simulink model "TorqueVect"  (Simulink 10.1)
settings: Solver=ode45  StartTime=0.0  StopTime=inf  RelTol=1e-3  EnableMultiTasking=on
undefined symbols (not defined in the file or in its folder): TC_Decr_Gas, TC_Derivative, TC_Incr_Gas, TC_On, TC_Relay_Off, TC_Relay_On, TV_On, TV_Override
libraries: CarMaker4SL x33, simulink x5, simulink_extras x4
(part 3 of 3)

== system TorqueVect/CarMaker/IPG Vehicle/PowerTrain/PTControl Example/PTControl_In/CreateBus PTC GearBoxM_In1 ==
  In : Inport
  BusCreator : BusCreator  Inputs=20
  Demux : Demux  Outputs=20
      settings: DisplayOption=none
  Out : Outport  VectorParamsAs1DForOutWhenUnconnected=off
  wires:
  In/1 -> Demux/1
  BusCreator/1 -> Out/1
  Demux/1 -> BusCreator/1  "PTC GearBoxM_In1 GearNo"
  Demux/2 -> BusCreator/2  "PTC GearBoxM_In1 GearNo_dis"
  Demux/3 -> BusCreator/3  "PTC GearBoxM_In1 Trq_DriveSrc_trg"
  Demux/4 -> BusCreator/4  "PTC GearBoxM_In1 i"
  Demux/5 -> BusCreator/5  "PTC GearBoxM_In1 rotv_in"
  Demux/6 -> BusCreator/6  "PTC GearBoxM_In1 rotv_out"
  Demux/7 -> BusCreator/7  "PTC GearBoxM_In1 Trq_in"
  Demux/8 -> BusCreator/8  "PTC GearBoxM_In1 Trq_out"
  Demux/9 -> BusCreator/9  "PTC GearBoxM_In1 Clutch Pos"
  Demux/10 -> BusCreator/10  "PTC GearBoxM_In1 Clutch rotv_in"
  Demux/11 -> BusCreator/11  "PTC GearBoxM_In1 Clutch rotv_out"
  Demux/12 -> BusCreator/12  "PTC GearBoxM_In1 Clutch Trq_in"
  Demux/13 -> BusCreator/13  "PTC GearBoxM_In1 Clutch Trq_out"
  Demux/14 -> BusCreator/14  "PTC GearBoxM_In1 Clutch i_TrqIn2Out"
  Demux/15 -> BusCreator/15  "PTC GearBoxM_In1 Clutch_dis Pos"
  Demux/16 -> BusCreator/16  "PTC GearBoxM_In1 Clutch_dis rotv_in"
  Demux/17 -> BusCreator/17  "PTC GearBoxM_In1 Clutch_dis rotv_out"
  Demux/18 -> BusCreator/18  "PTC GearBoxM_In1 Clutch_dis Trq_in"
  Demux/19 -> BusCreator/19  "PTC GearBoxM_In1 Clutch_dis Trq_out"
  Demux/20 -> BusCreator/20  "PTC GearBoxM_In1 Clutch_dis i_TrqIn2Out"

== system TorqueVect/CarMaker/IPG Vehicle/PowerTrain/PTControl Example/PTControl_In/CreateBus PTC GearBoxM_In2 ==
  In : Inport
  BusCreator : BusCreator  Inputs=20
  Demux : Demux  Outputs=20
      settings: DisplayOption=none
  Out : Outport  VectorParamsAs1DForOutWhenUnconnected=off
  wires:
  In/1 -> Demux/1
  BusCreator/1 -> Out/1
  Demux/1 -> BusCreator/1  "PTC GearBoxM_In2 GearNo"
  Demux/2 -> BusCreator/2  "PTC GearBoxM_In2 GearNo_dis"
  Demux/3 -> BusCreator/3  "PTC GearBoxM_In2 Trq_DriveSrc_trg"
  Demux/4 -> BusCreator/4  "PTC GearBoxM_In2 i"
  Demux/5 -> BusCreator/5  "PTC GearBoxM_In2 rotv_in"
  Demux/6 -> BusCreator/6  "PTC GearBoxM_In2 rotv_out"
  Demux/7 -> BusCreator/7  "PTC GearBoxM_In2 Trq_in"
  Demux/8 -> BusCreator/8  "PTC GearBoxM_In2 Trq_out"
  Demux/9 -> BusCreator/9  "PTC GearBoxM_In2 Clutch Pos"
  Demux/10 -> BusCreator/10  "PTC GearBoxM_In2 Clutch rotv_in"
  Demux/11 -> BusCreator/11  "PTC GearBoxM_In2 Clutch rotv_out"
  Demux/12 -> BusCreator/12  "PTC GearBoxM_In2 Clutch Trq_in"
  Demux/13 -> BusCreator/13  "PTC GearBoxM_In2 Clutch Trq_out"
  Demux/14 -> BusCreator/14  "PTC GearBoxM_In2 Clutch i_TrqIn2Out"
  Demux/15 -> BusCreator/15  "PTC GearBoxM_In2 Clutch_dis Pos"
  Demux/16 -> BusCreator/16  "PTC GearBoxM_In2 Clutch_dis rotv_in"
  Demux/17 -> BusCreator/17  "PTC GearBoxM_In2 Clutch_dis rotv_out"
  Demux/18 -> BusCreator/18  "PTC GearBoxM_In2 Clutch_dis Trq_in"
  Demux/19 -> BusCreator/19  "PTC GearBoxM_In2 Clutch_dis Trq_out"
  Demux/20 -> BusCreator/20  "PTC GearBoxM_In2 Clutch_dis i_TrqIn2Out"

== system TorqueVect/CarMaker/IPG Vehicle/PowerTrain/PTControl Example/PTControl_In/CreateBus PTC GearBoxM_In3 ==
  In : Inport
  BusCreator : BusCreator  Inputs=20
  Demux : Demux  Outputs=20
      settings: DisplayOption=none
  Out : Outport  VectorParamsAs1DForOutWhenUnconnected=off
  wires:
  In/1 -> Demux/1
  BusCreator/1 -> Out/1
  Demux/1 -> BusCreator/1  "PTC GearBoxM_In3 GearNo"
  Demux/2 -> BusCreator/2  "PTC GearBoxM_In3 GearNo_dis"
  Demux/3 -> BusCreator/3  "PTC GearBoxM_In3 Trq_DriveSrc_trg"
  Demux/4 -> BusCreator/4  "PTC GearBoxM_In3 i"
  Demux/5 -> BusCreator/5  "PTC GearBoxM_In3 rotv_in"
  Demux/6 -> BusCreator/6  "PTC GearBoxM_In3 rotv_out"
  Demux/7 -> BusCreator/7  "PTC GearBoxM_In3 Trq_in"
  Demux/8 -> BusCreator/8  "PTC GearBoxM_In3 Trq_out"
  Demux/9 -> BusCreator/9  "PTC GearBoxM_In3 Clutch Pos"
  Demux/10 -> BusCreator/10  "PTC GearBoxM_In3 Clutch rotv_in"
  Demux/11 -> BusCreator/11  "PTC GearBoxM_In3 Clutch rotv_out"
  Demux/12 -> BusCreator/12  "PTC GearBoxM_In3 Clutch Trq_in"
  Demux/13 -> BusCreator/13  "PTC GearBoxM_In3 Clutch Trq_out"
  Demux/14 -> BusCreator/14  "PTC GearBoxM_In3 Clutch i_TrqIn2Out"
  Demux/15 -> BusCreator/15  "PTC GearBoxM_In3 Clutch_dis Pos"
  Demux/16 -> BusCreator/16  "PTC GearBoxM_In3 Clutch_dis rotv_in"
  Demux/17 -> BusCreator/17  "PTC GearBoxM_In3 Clutch_dis rotv_out"
  Demux/18 -> BusCreator/18  "PTC GearBoxM_In3 Clutch_dis Trq_in"
  Demux/19 -> BusCreator/19  "PTC GearBoxM_In3 Clutch_dis Trq_out"
  Demux/20 -> BusCreator/20  "PTC GearBoxM_In3 Clutch_dis i_TrqIn2Out"

== system TorqueVect/CarMaker/IPG Vehicle/PowerTrain/PTControl Example/PTControl_In/CreateBus PTC ISGIn ==
  In : Inport
  BusCreator : BusCreator  Inputs=9
  Demux : Demux  Outputs=9
      settings: DisplayOption=none
  Out : Outport  VectorParamsAs1DForOutWhenUnconnected=off
  wires:
  In/1 -> Demux/1
  BusCreator/1 -> Out/1
  Demux/1 -> BusCreator/1  "PTC ISGIn rotv"
  Demux/2 -> BusCreator/2  "PTC ISGIn Trq"
  Demux/3 -> BusCreator/3  "PTC ISGIn TrqMot_max"
  Demux/4 -> BusCreator/4  "PTC ISGIn TrqGen_max"
  Demux/5 -> BusCreator/5  "PTC ISGIn PwrElec"
  Demux/6 -> BusCreator/6  "PTC ISGIn i_M2W_FL"
  Demux/7 -> BusCreator/7  "PTC ISGIn i_M2W_FR"
  Demux/8 -> BusCreator/8  "PTC ISGIn i_M2W_RL"
  Demux/9 -> BusCreator/9  "PTC ISGIn i_M2W_RR"

== system TorqueVect/CarMaker/IPG Vehicle/PowerTrain/PTControl Example/PTControl_In/CreateBus PTC MotorIn0 ==
  In : Inport
  BusCreator : BusCreator  Inputs=9
  Demux : Demux  Outputs=9
      settings: DisplayOption=none
  Out : Outport  VectorParamsAs1DForOutWhenUnconnected=off
  wires:
  In/1 -> Demux/1
  BusCreator/1 -> Out/1
  Demux/1 -> BusCreator/1  "PTC MotorIn0 rotv"
  Demux/2 -> BusCreator/2  "PTC MotorIn0 Trq"
  Demux/3 -> BusCreator/3  "PTC MotorIn0 TrqMot_max"
  Demux/4 -> BusCreator/4  "PTC MotorIn0 TrqGen_max"
  Demux/5 -> BusCreator/5  "PTC MotorIn0 PwrElec"
  Demux/6 -> BusCreator/6  "PTC MotorIn0 i_M2W_FL"
  Demux/7 -> BusCreator/7  "PTC MotorIn0 i_M2W_FR"
  Demux/8 -> BusCreator/8  "PTC MotorIn0 i_M2W_RL"
  Demux/9 -> BusCreator/9  "PTC MotorIn0 i_M2W_RR"

== system TorqueVect/CarMaker/IPG Vehicle/PowerTrain/PTControl Example/PTControl_In/CreateBus PTC MotorIn1 ==
  In : Inport
  BusCreator : BusCreator  Inputs=9
  Demux : Demux  Outputs=9
      settings: DisplayOption=none
  Out : Outport  VectorParamsAs1DForOutWhenUnconnected=off
  wires:
  In/1 -> Demux/1
  BusCreator/1 -> Out/1
  Demux/1 -> BusCreator/1  "PTC MotorIn1 rotv"
  Demux/2 -> BusCreator/2  "PTC MotorIn1 Trq"
  Demux/3 -> BusCreator/3  "PTC MotorIn1 TrqMot_max"
  Demux/4 -> BusCreator/4  "PTC MotorIn1 TrqGen_max"
  Demux/5 -> BusCreator/5  "PTC MotorIn1 PwrElec"
  Demux/6 -> BusCreator/6  "PTC MotorIn1 i_M2W_FL"
  Demux/7 -> BusCreator/7  "PTC MotorIn1 i_M2W_FR"
  Demux/8 -> BusCreator/8  "PTC MotorIn1 i_M2W_RL"
  Demux/9 -> BusCreator/9  "PTC MotorIn1 i_M2W_RR"

== system TorqueVect/CarMaker/IPG Vehicle/PowerTrain/PTControl Example/PTControl_In/CreateBus PTC MotorIn2 ==
  In : Inport
  BusCreator : BusCreator  Inputs=9
  Demux : Demux  Outputs=9
      settings: DisplayOption=none
  Out : Outport  VectorParamsAs1DForOutWhenUnconnected=off
  wires:
  In/1 -> Demux/1
  BusCreator/1 -> Out/1
  Demux/1 -> BusCreator/1  "PTC MotorIn2 rotv"
  Demux/2 -> BusCreator/2  "PTC MotorIn2 Trq"
  Demux/3 -> BusCreator/3  "PTC MotorIn2 TrqMot_max"
  Demux/4 -> BusCreator/4  "PTC MotorIn2 TrqGen_max"
  Demux/5 -> BusCreator/5  "PTC MotorIn2 PwrElec"
  Demux/6 -> BusCreator/6  "PTC MotorIn2 i_M2W_FL"
  Demux/7 -> BusCreator/7  "PTC MotorIn2 i_M2W_FR"
  Demux/8 -> BusCreator/8  "PTC MotorIn2 i_M2W_RL"
  Demux/9 -> BusCreator/9  "PTC MotorIn2 i_M2W_RR"

== system TorqueVect/CarMaker/IPG Vehicle/PowerTrain/PTControl Example/PTControl_In/CreateBus PTC MotorIn3 ==
  In : Inport
  BusCreator : BusCreator  Inputs=9
  Demux : Demux  Outputs=9
      settings: DisplayOption=none
  Out : Outport  VectorParamsAs1DForOutWhenUnconnected=off
  wires:
  In/1 -> Demux/1
  BusCreator/1 -> Out/1
  Demux/1 -> BusCreator/1  "PTC MotorIn3 rotv"
  Demux/2 -> BusCreator/2  "PTC MotorIn3 Trq"
  Demux/3 -> BusCreator/3  "PTC MotorIn3 TrqMot_max"
  Demux/4 -> BusCreator/4  "PTC MotorIn3 TrqGen_max"
  Demux/5 -> BusCreator/5  "PTC MotorIn3 PwrElec"
  Demux/6 -> BusCreator/6  "PTC MotorIn3 i_M2W_FL"
  Demux/7 -> BusCreator/7  "PTC MotorIn3 i_M2W_FR"
  Demux/8 -> BusCreator/8  "PTC MotorIn3 i_M2W_RL"
  Demux/9 -> BusCreator/9  "PTC MotorIn3 i_M2W_RR"

== system TorqueVect/CarMaker/IPG Vehicle/PowerTrain/PTControl Example/PTControl_In/CreateBus PTC PwrSupplyIn ==
  In : Inport
  BusCreator : BusCreator  Inputs=12
  Demux : Demux  Outputs=12
      settings: DisplayOption=none
  Out : Outport  VectorParamsAs1DForOutWhenUnconnected=off
  wires:
  In/1 -> Demux/1
  BusCreator/1 -> Out/1
  Demux/1 -> BusCreator/1  "PTC PwrSupplyIn Pwr_LV"
  Demux/2 -> BusCreator/2  "PTC PwrSupplyIn Pwr_HV1"
  Demux/3 -> BusCreator/3  "PTC PwrSupplyIn Pwr_HV2"
  Demux/4 -> BusCreator/4  "PTC PwrSupplyIn Voltage_LV"
  Demux/5 -> BusCreator/5  "PTC PwrSupplyIn Voltage_HV1"
  Demux/6 -> BusCreator/6  "PTC PwrSupplyIn Voltage_HV2"
  Demux/7 -> BusCreator/7  "PTC PwrSupplyIn Pwr_HV1toLV"
  Demux/8 -> BusCreator/8  "PTC PwrSupplyIn Pwr_HV1toHV2"
  Demux/9 -> BusCreator/9  "PTC PwrSupplyIn Pwr_HV1toLV_max"
  Demux/10 -> BusCreator/10  "PTC PwrSupplyIn Pwr_HV1toHV2_max"
  Demux/11 -> BusCreator/11  "PTC PwrSupplyIn Eta_HV1toLV"
  Demux/12 -> BusCreator/12  "PTC PwrSupplyIn Eta_HV1toHV2"

== system TorqueVect/CarMaker/IPG Vehicle/PowerTrain/PTControl Example/PTControl_In/CreateBus PTC Vehicle Ctrl ==
  In : Inport
  BusCreator : BusCreator  Inputs=8
  Demux : Demux  Outputs=8
      settings: DisplayOption=none
  Out : Outport  VectorParamsAs1DForOutWhenUnconnected=off
  wires:
  In/1 -> Demux/1
  BusCreator/1 -> Out/1
  Demux/1 -> BusCreator/1  "PTC Key"
  Demux/2 -> BusCreator/2  "PTC SST"
  Demux/3 -> BusCreator/3  "PTC SelectorCtrl"
  Demux/4 -> BusCreator/4  "PTC GearNoTrg"
  Demux/5 -> BusCreator/5  "PTC Clutch"
  Demux/6 -> BusCreator/6  "PTC Gas"
  Demux/7 -> BusCreator/7  "PTC Brake"
  Demux/8 -> BusCreator/8  "PTC Velocity"

== system TorqueVect/CarMaker/IPG Vehicle/PowerTrain/PTControl Example/PTControl_In/CreateBus PTC WheelIn ==
  In : Inport
  BusCreator : BusCreator  Inputs=4
  Demux : Demux
      settings: DisplayOption=none
  Out : Outport  VectorParamsAs1DForOutWhenUnconnected=off
  wires:
  In/1 -> Demux/1
  BusCreator/1 -> Out/1
  Demux/1 -> BusCreator/1  "PTC WheelIn_FL Trq_BrakeReg_trg"
  Demux/2 -> BusCreator/2  "PTC WheelIn_FR Trq_BrakeReg_trg"
  Demux/3 -> BusCreator/3  "PTC WheelIn_RL Trq_BrakeReg_trg"
  Demux/4 -> BusCreator/4  "PTC WheelIn_RR Trq_BrakeReg_trg"

== system TorqueVect/CarMaker/IPG Vehicle/PowerTrain/PTControl Example/PTControl_In/CreateBus PTC_Cfg Battery ==
  In : Inport
  BusCreator : BusCreator  Inputs=8
  Demux : Demux  Outputs=8
      settings: DisplayOption=none
  Out : Outport  VectorParamsAs1DForOutWhenUnconnected=off
  wires:
  In/1 -> Demux/1
  BusCreator/1 -> Out/1
  Demux/1 -> BusCreator/1  "PTC_Cfg BattLV SOC_min"
  Demux/2 -> BusCreator/2  "PTC_Cfg BattLV SOC_max"
  Demux/3 -> BusCreator/3  "PTC_Cfg BattLV Capacity"
  Demux/4 -> BusCreator/4  "PTC_Cfg BattLV Voltage"
  Demux/5 -> BusCreator/5  "PTC_Cfg BattHV SOC_min"
  Demux/6 -> BusCreator/6  "PTC_Cfg BattHV SOC_max"
  Demux/7 -> BusCreator/7  "PTC_Cfg BattHV Capacity"
  Demux/8 -> BusCreator/8  "PTC_Cfg BattHV Voltage"

== system TorqueVect/CarMaker/IPG Vehicle/PowerTrain/PTControl Example/PTControl_In/CreateBus PTC_Cfg Engine ==
  In : Inport
  BusCreator : BusCreator  Inputs=4
  Demux : Demux
      settings: DisplayOption=none
  Out : Outport  VectorParamsAs1DForOutWhenUnconnected=off
  wires:
  In/1 -> Demux/1
  BusCreator/1 -> Out/1
  Demux/1 -> BusCreator/1  "PTC_Cfg Engine Fuel_l2kWh"
  Demux/2 -> BusCreator/2  "PTC_Cfg Engine rotv_max"
  Demux/3 -> BusCreator/3  "PTC_Cfg Engine rotv_idle"
  Demux/4 -> BusCreator/4  "PTC_Cfg Engine rotv_opt"

== system TorqueVect/CarMaker/IPG Vehicle/PowerTrain/PTControl Example/PTControl_In/CreateBus PTC_Cfg GearBox ==
  In : Inport
  BusCreator : BusCreator  Inputs=38
  Demux : Demux  Outputs=38
      settings: DisplayOption=none
  Out : Outport  VectorParamsAs1DForOutWhenUnconnected=off
  wires:
  In/1 -> Demux/1
  BusCreator/1 -> Out/1
  Demux/1 -> BusCreator/1  "PTC_Cfg GearBox GBKind"
  Demux/2 -> BusCreator/2  "PTC_Cfg GearBox ClKind"
  Demux/3 -> BusCreator/3  "PTC_Cfg GearBox nFGears"
  Demux/4 -> BusCreator/4  "PTC_Cfg GearBox iFGear0"
  Demux/5 -> BusCreator/5  "PTC_Cfg GearBox iFGear1"
  Demux/6 -> BusCreator/6  "PTC_Cfg GearBox iFGear2"
  Demux/7 -> BusCreator/7  "PTC_Cfg GearBox iFGear3"
  Demux/8 -> BusCreator/8  "PTC_Cfg GearBox iFGear4"
  Demux/9 -> BusCreator/9  "PTC_Cfg GearBox iFGear5"
  Demux/10 -> BusCreator/10  "PTC_Cfg GearBox iFGear6"
  Demux/11 -> BusCreator/11  "PTC_Cfg GearBox iFGear7"
  Demux/12 -> BusCreator/12  "PTC_Cfg GearBox iFGear8"
  Demux/13 -> BusCreator/13  "PTC_Cfg GearBox iFGear9"
  Demux/14 -> BusCreator/14  "PTC_Cfg GearBox iFGear10"
  Demux/15 -> BusCreator/15  "PTC_Cfg GearBox iFGear11"
  Demux/16 -> BusCreator/16  "PTC_Cfg GearBox iFGear12"
  Demux/17 -> BusCreator/17  "PTC_Cfg GearBox iFGear13"
  Demux/18 -> BusCreator/18  "PTC_Cfg GearBox iFGear14"
  Demux/19 -> BusCreator/19  "PTC_Cfg GearBox iFGear15"
  Demux/20 -> BusCreator/20  "PTC_Cfg GearBox iFGear16"
  Demux/21 -> BusCreator/21  "PTC_Cfg GearBox nBGears"
  Demux/22 -> BusCreator/22  "PTC_Cfg GearBox iBGear0"
  Demux/23 -> BusCreator/23  "PTC_Cfg GearBox iBGear1"
  Demux/24 -> BusCreator/24  "PTC_Cfg GearBox iBGear2"
  Demux/25 -> BusCreator/25  "PTC_Cfg GearBox iBGear3"
  Demux/26 -> BusCreator/26  "PTC_Cfg GearBox iBGear4"
  Demux/27 -> BusCreator/27  "PTC_Cfg GearBox iBGear5"
  Demux/28 -> BusCreator/28  "PTC_Cfg GearBox iBGear6"
  Demux/29 -> BusCreator/29  "PTC_Cfg GearBox iBGear7"
  Demux/30 -> BusCreator/30  "PTC_Cfg GearBox iBGear8"
  Demux/31 -> BusCreator/31  "PTC_Cfg GearBox iBGear9"
  Demux/32 -> BusCreator/32  "PTC_Cfg GearBox iBGear10"
  Demux/33 -> BusCreator/33  "PTC_Cfg GearBox iBGear11"
  Demux/34 -> BusCreator/34  "PTC_Cfg GearBox iBGear12"
  Demux/35 -> BusCreator/35  "PTC_Cfg GearBox iBGear13"
  Demux/36 -> BusCreator/36  "PTC_Cfg GearBox iBGear14"
  Demux/37 -> BusCreator/37  "PTC_Cfg GearBox iBGear15"
  Demux/38 -> BusCreator/38  "PTC_Cfg GearBox iBGear16"

== system TorqueVect/CarMaker/IPG Vehicle/PowerTrain/PTControl Example/PTControl_In/CreateBus PTC_Cfg GearBoxM0 ==
  In : Inport
  BusCreator : BusCreator  Inputs=38
  Demux : Demux  Outputs=38
      settings: DisplayOption=none
  Out : Outport  VectorParamsAs1DForOutWhenUnconnected=off
  wires:
  In/1 -> Demux/1
  BusCreator/1 -> Out/1
  Demux/1 -> BusCreator/1  "PTC_Cfg GearBoxM0 GBKind"
  Demux/2 -> BusCreator/2  "PTC_Cfg GearBoxM0 ClKind"
  Demux/3 -> BusCreator/3  "PTC_Cfg GearBoxM0 nFGears"
  Demux/4 -> BusCreator/4  "PTC_Cfg GearBoxM0 iFGear0"
  Demux/5 -> BusCreator/5  "PTC_Cfg GearBoxM0 iFGear1"
  Demux/6 -> BusCreator/6  "PTC_Cfg GearBoxM0 iFGear2"
  Demux/7 -> BusCreator/7  "PTC_Cfg GearBoxM0 iFGear3"
  Demux/8 -> BusCreator/8  "PTC_Cfg GearBoxM0 iFGear4"
  Demux/9 -> BusCreator/9  "PTC_Cfg GearBoxM0 iFGear5"
  Demux/10 -> BusCreator/10  "PTC_Cfg GearBoxM0 iFGear6"
  Demux/11 -> BusCreator/11  "PTC_Cfg GearBoxM0 iFGear7"
  Demux/12 -> BusCreator/12  "PTC_Cfg GearBoxM0 iFGear8"
  Demux/13 -> BusCreator/13  "PTC_Cfg GearBoxM0 iFGear9"
  Demux/14 -> BusCreator/14  "PTC_Cfg GearBoxM0 iFGear10"
  Demux/15 -> BusCreator/15  "PTC_Cfg GearBoxM0 iFGear11"
  Demux/16 -> BusCreator/16  "PTC_Cfg GearBoxM0 iFGear12"
  Demux/17 -> BusCreator/17  "PTC_Cfg GearBoxM0 iFGear13"
  Demux/18 -> BusCreator/18  "PTC_Cfg GearBoxM0 iFGear14"
  Demux/19 -> BusCreator/19  "PTC_Cfg GearBoxM0 iFGear15"
  Demux/20 -> BusCreator/20  "PTC_Cfg GearBoxM0 iFGear16"
  Demux/21 -> BusCreator/21  "PTC_Cfg GearBoxM0 nBGears"
  Demux/22 -> BusCreator/22  "PTC_Cfg GearBoxM0 iBGear0"
  Demux/23 -> BusCreator/23  "PTC_Cfg GearBoxM0 iBGear1"
  Demux/24 -> BusCreator/24  "PTC_Cfg GearBoxM0 iBGear2"
  Demux/25 -> BusCreator/25  "PTC_Cfg GearBoxM0 iBGear3"
  Demux/26 -> BusCreator/26  "PTC_Cfg GearBoxM0 iBGear4"
  Demux/27 -> BusCreator/27  "PTC_Cfg GearBoxM0 iBGear5"
  Demux/28 -> BusCreator/28  "PTC_Cfg GearBoxM0 iBGear6"
  Demux/29 -> BusCreator/29  "PTC_Cfg GearBoxM0 iBGear7"
  Demux/30 -> BusCreator/30  "PTC_Cfg GearBoxM0 iBGear8"
  Demux/31 -> BusCreator/31  "PTC_Cfg GearBoxM0 iBGear9"
  Demux/32 -> BusCreator/32  "PTC_Cfg GearBoxM0 iBGear10"
  Demux/33 -> BusCreator/33  "PTC_Cfg GearBoxM0 iBGear11"
  Demux/34 -> BusCreator/34  "PTC_Cfg GearBoxM0 iBGear12"
  Demux/35 -> BusCreator/35  "PTC_Cfg GearBoxM0 iBGear13"
  Demux/36 -> BusCreator/36  "PTC_Cfg GearBoxM0 iBGear14"
  Demux/37 -> BusCreator/37  "PTC_Cfg GearBoxM0 iBGear15"
  Demux/38 -> BusCreator/38  "PTC_Cfg GearBoxM0 iBGear16"

== system TorqueVect/CarMaker/IPG Vehicle/PowerTrain/PTControl Example/PTControl_In/CreateBus PTC_Cfg GearBoxM1 ==
  In : Inport
  BusCreator : BusCreator  Inputs=38
  Demux : Demux  Outputs=38
      settings: DisplayOption=none
  Out : Outport  VectorParamsAs1DForOutWhenUnconnected=off
  wires:
  In/1 -> Demux/1
  BusCreator/1 -> Out/1
  Demux/1 -> BusCreator/1  "PTC_Cfg GearBoxM1 GBKind"
  Demux/2 -> BusCreator/2  "PTC_Cfg GearBoxM1 ClKind"
  Demux/3 -> BusCreator/3  "PTC_Cfg GearBoxM1 nFGears"
  Demux/4 -> BusCreator/4  "PTC_Cfg GearBoxM1 iFGear0"
  Demux/5 -> BusCreator/5  "PTC_Cfg GearBoxM1 iFGear1"
  Demux/6 -> BusCreator/6  "PTC_Cfg GearBoxM1 iFGear2"
  Demux/7 -> BusCreator/7  "PTC_Cfg GearBoxM1 iFGear3"
  Demux/8 -> BusCreator/8  "PTC_Cfg GearBoxM1 iFGear4"
  Demux/9 -> BusCreator/9  "PTC_Cfg GearBoxM1 iFGear5"
  Demux/10 -> BusCreator/10  "PTC_Cfg GearBoxM1 iFGear6"
  Demux/11 -> BusCreator/11  "PTC_Cfg GearBoxM1 iFGear7"
  Demux/12 -> BusCreator/12  "PTC_Cfg GearBoxM1 iFGear8"
  Demux/13 -> BusCreator/13  "PTC_Cfg GearBoxM1 iFGear9"
  Demux/14 -> BusCreator/14  "PTC_Cfg GearBoxM1 iFGear10"
  Demux/15 -> BusCreator/15  "PTC_Cfg GearBoxM1 iFGear11"
  Demux/16 -> BusCreator/16  "PTC_Cfg GearBoxM1 iFGear12"
  Demux/17 -> BusCreator/17  "PTC_Cfg GearBoxM1 iFGear13"
  Demux/18 -> BusCreator/18  "PTC_Cfg GearBoxM1 iFGear14"
  Demux/19 -> BusCreator/19  "PTC_Cfg GearBoxM1 iFGear15"
  Demux/20 -> BusCreator/20  "PTC_Cfg GearBoxM1 iFGear16"
  Demux/21 -> BusCreator/21  "PTC_Cfg GearBoxM1 nBGears"
  Demux/22 -> BusCreator/22  "PTC_Cfg GearBoxM1 iBGear0"
  Demux/23 -> BusCreator/23  "PTC_Cfg GearBoxM1 iBGear1"
  Demux/24 -> BusCreator/24  "PTC_Cfg GearBoxM1 iBGear2"
  Demux/25 -> BusCreator/25  "PTC_Cfg GearBoxM1 iBGear3"
  Demux/26 -> BusCreator/26  "PTC_Cfg GearBoxM1 iBGear4"
  Demux/27 -> BusCreator/27  "PTC_Cfg GearBoxM1 iBGear5"
  Demux/28 -> BusCreator/28  "PTC_Cfg GearBoxM1 iBGear6"
  Demux/29 -> BusCreator/29  "PTC_Cfg GearBoxM1 iBGear7"
  Demux/30 -> BusCreator/30  "PTC_Cfg GearBoxM1 iBGear8"
  Demux/31 -> BusCreator/31  "PTC_Cfg GearBoxM1 iBGear9"
  Demux/32 -> BusCreator/32  "PTC_Cfg GearBoxM1 iBGear10"
  Demux/33 -> BusCreator/33  "PTC_Cfg GearBoxM1 iBGear11"
  Demux/34 -> BusCreator/34  "PTC_Cfg GearBoxM1 iBGear12"
  Demux/35 -> BusCreator/35  "PTC_Cfg GearBoxM1 iBGear13"
  Demux/36 -> BusCreator/36  "PTC_Cfg GearBoxM1 iBGear14"
  Demux/37 -> BusCreator/37  "PTC_Cfg GearBoxM1 iBGear15"
  Demux/38 -> BusCreator/38  "PTC_Cfg GearBoxM1 iBGear16"

== system TorqueVect/CarMaker/IPG Vehicle/PowerTrain/PTControl Example/PTControl_In/CreateBus PTC_Cfg GearBoxM2 ==
  In : Inport
  BusCreator : BusCreator  Inputs=38
  Demux : Demux  Outputs=38
      settings: DisplayOption=none
  Out : Outport  VectorParamsAs1DForOutWhenUnconnected=off
  wires:
  In/1 -> Demux/1
  BusCreator/1 -> Out/1
  Demux/1 -> BusCreator/1  "PTC_Cfg GearBoxM2 GBKind"
  Demux/2 -> BusCreator/2  "PTC_Cfg GearBoxM2 ClKind"
  Demux/3 -> BusCreator/3  "PTC_Cfg GearBoxM2 nFGears"
  Demux/4 -> BusCreator/4  "PTC_Cfg GearBoxM2 iFGear0"
  Demux/5 -> BusCreator/5  "PTC_Cfg GearBoxM2 iFGear1"
  Demux/6 -> BusCreator/6  "PTC_Cfg GearBoxM2 iFGear2"
  Demux/7 -> BusCreator/7  "PTC_Cfg GearBoxM2 iFGear3"
  Demux/8 -> BusCreator/8  "PTC_Cfg GearBoxM2 iFGear4"
  Demux/9 -> BusCreator/9  "PTC_Cfg GearBoxM2 iFGear5"
  Demux/10 -> BusCreator/10  "PTC_Cfg GearBoxM2 iFGear6"
  Demux/11 -> BusCreator/11  "PTC_Cfg GearBoxM2 iFGear7"
  Demux/12 -> BusCreator/12  "PTC_Cfg GearBoxM2 iFGear8"
  Demux/13 -> BusCreator/13  "PTC_Cfg GearBoxM2 iFGear9"
  Demux/14 -> BusCreator/14  "PTC_Cfg GearBoxM2 iFGear10"
  Demux/15 -> BusCreator/15  "PTC_Cfg GearBoxM2 iFGear11"
  Demux/16 -> BusCreator/16  "PTC_Cfg GearBoxM2 iFGear12"
  Demux/17 -> BusCreator/17  "PTC_Cfg GearBoxM2 iFGear13"
  Demux/18 -> BusCreator/18  "PTC_Cfg GearBoxM2 iFGear14"
  Demux/19 -> BusCreator/19  "PTC_Cfg GearBoxM2 iFGear15"
  Demux/20 -> BusCreator/20  "PTC_Cfg GearBoxM2 iFGear16"
  Demux/21 -> BusCreator/21  "PTC_Cfg GearBoxM2 nBGears"
  Demux/22 -> BusCreator/22  "PTC_Cfg GearBoxM2 iBGear0"
  Demux/23 -> BusCreator/23  "PTC_Cfg GearBoxM2 iBGear1"
  Demux/24 -> BusCreator/24  "PTC_Cfg GearBoxM2 iBGear2"
  Demux/25 -> BusCreator/25  "PTC_Cfg GearBoxM2 iBGear3"
  Demux/26 -> BusCreator/26  "PTC_Cfg GearBoxM2 iBGear4"
  Demux/27 -> BusCreator/27  "PTC_Cfg GearBoxM2 iBGear5"
  Demux/28 -> BusCreator/28  "PTC_Cfg GearBoxM2 iBGear6"
  Demux/29 -> BusCreator/29  "PTC_Cfg GearBoxM2 iBGear7"
  Demux/30 -> BusCreator/30  "PTC_Cfg GearBoxM2 iBGear8"
  Demux/31 -> BusCreator/31  "PTC_Cfg GearBoxM2 iBGear9"
  Demux/32 -> BusCreator/32  "PTC_Cfg GearBoxM2 iBGear10"
  Demux/33 -> BusCreator/33  "PTC_Cfg GearBoxM2 iBGear11"
  Demux/34 -> BusCreator/34  "PTC_Cfg GearBoxM2 iBGear12"
  Demux/35 -> BusCreator/35  "PTC_Cfg GearBoxM2 iBGear13"
  Demux/36 -> BusCreator/36  "PTC_Cfg GearBoxM2 iBGear14"
  Demux/37 -> BusCreator/37  "PTC_Cfg GearBoxM2 iBGear15"
  Demux/38 -> BusCreator/38  "PTC_Cfg GearBoxM2 iBGear16"

== system TorqueVect/CarMaker/IPG Vehicle/PowerTrain/PTControl Example/PTControl_In/CreateBus PTC_Cfg GearBoxM3 ==
  In : Inport
  BusCreator : BusCreator  Inputs=38
  Demux : Demux  Outputs=38
      settings: DisplayOption=none
  Out : Outport  VectorParamsAs1DForOutWhenUnconnected=off
  wires:
  In/1 -> Demux/1
  BusCreator/1 -> Out/1
  Demux/1 -> BusCreator/1  "PTC_Cfg GearBoxM3 GBKind"
  Demux/2 -> BusCreator/2  "PTC_Cfg GearBoxM3 ClKind"
  Demux/3 -> BusCreator/3  "PTC_Cfg GearBoxM3 nFGears"
  Demux/4 -> BusCreator/4  "PTC_Cfg GearBoxM3 iFGear0"
  Demux/5 -> BusCreator/5  "PTC_Cfg GearBoxM3 iFGear1"
  Demux/6 -> BusCreator/6  "PTC_Cfg GearBoxM3 iFGear2"
  Demux/7 -> BusCreator/7  "PTC_Cfg GearBoxM3 iFGear3"
  Demux/8 -> BusCreator/8  "PTC_Cfg GearBoxM3 iFGear4"
  Demux/9 -> BusCreator/9  "PTC_Cfg GearBoxM3 iFGear5"
  Demux/10 -> BusCreator/10  "PTC_Cfg GearBoxM3 iFGear6"
  Demux/11 -> BusCreator/11  "PTC_Cfg GearBoxM3 iFGear7"
  Demux/12 -> BusCreator/12  "PTC_Cfg GearBoxM3 iFGear8"
  Demux/13 -> BusCreator/13  "PTC_Cfg GearBoxM3 iFGear9"
  Demux/14 -> BusCreator/14  "PTC_Cfg GearBoxM3 iFGear10"
  Demux/15 -> BusCreator/15  "PTC_Cfg GearBoxM3 iFGear11"
  Demux/16 -> BusCreator/16  "PTC_Cfg GearBoxM3 iFGear12"
  Demux/17 -> BusCreator/17  "PTC_Cfg GearBoxM3 iFGear13"
  Demux/18 -> BusCreator/18  "PTC_Cfg GearBoxM3 iFGear14"
  Demux/19 -> BusCreator/19  "PTC_Cfg GearBoxM3 iFGear15"
  Demux/20 -> BusCreator/20  "PTC_Cfg GearBoxM3 iFGear16"
  Demux/21 -> BusCreator/21  "PTC_Cfg GearBoxM3 nBGears"
  Demux/22 -> BusCreator/22  "PTC_Cfg GearBoxM3 iBGear0"
  Demux/23 -> BusCreator/23  "PTC_Cfg GearBoxM3 iBGear1"
  Demux/24 -> BusCreator/24  "PTC_Cfg GearBoxM3 iBGear2"
  Demux/25 -> BusCreator/25  "PTC_Cfg GearBoxM3 iBGear3"
  Demux/26 -> BusCreator/26  "PTC_Cfg GearBoxM3 iBGear4"
  Demux/27 -> BusCreator/27  "PTC_Cfg GearBoxM3 iBGear5"
  Demux/28 -> BusCreator/28  "PTC_Cfg GearBoxM3 iBGear6"
  Demux/29 -> BusCreator/29  "PTC_Cfg GearBoxM3 iBGear7"
  Demux/30 -> BusCreator/30  "PTC_Cfg GearBoxM3 iBGear8"
  Demux/31 -> BusCreator/31  "PTC_Cfg GearBoxM3 iBGear9"
  Demux/32 -> BusCreator/32  "PTC_Cfg GearBoxM3 iBGear10"
  Demux/33 -> BusCreator/33  "PTC_Cfg GearBoxM3 iBGear11"
  Demux/34 -> BusCreator/34  "PTC_Cfg GearBoxM3 iBGear12"
  Demux/35 -> BusCreator/35  "PTC_Cfg GearBoxM3 iBGear13"
  Demux/36 -> BusCreator/36  "PTC_Cfg GearBoxM3 iBGear14"
  Demux/37 -> BusCreator/37  "PTC_Cfg GearBoxM3 iBGear15"
  Demux/38 -> BusCreator/38  "PTC_Cfg GearBoxM3 iBGear16"

== system TorqueVect/CarMaker/IPG Vehicle/PowerTrain/PTControl Example/PTControl_In/CreateBus PTC_Cfg ISG ==
  In : Inport
  BusCreator : BusCreator  Inputs=4
  Demux : Demux
      settings: DisplayOption=none
  Out : Outport  VectorParamsAs1DForOutWhenUnconnected=off
  wires:
  In/1 -> Demux/1
  BusCreator/1 -> Out/1
  Demux/1 -> BusCreator/1  "PTC_Cfg ISG Level"
  Demux/2 -> BusCreator/2  "PTC_Cfg ISG Ratio"
  Demux/3 -> BusCreator/3  "PTC_Cfg ISG rotv_Mot_max"
  Demux/4 -> BusCreator/4  "PTC_Cfg ISG rotv_Gen_max"

== system TorqueVect/CarMaker/IPG Vehicle/PowerTrain/PTControl Example/PTControl_In/CreateBus PTC_Cfg Misc ==
  In : Inport
  BusCreator : BusCreator  Inputs=13
  Demux : Demux  Outputs=13
      settings: DisplayOption=none
  Out : Outport  VectorParamsAs1DForOutWhenUnconnected=off
  wires:
  In/1 -> Demux/1
  BusCreator/1 -> Out/1
  Demux/1 -> BusCreator/1  "PTC_Cfg PTKind"
  Demux/2 -> BusCreator/2  "PTC_Cfg ClKind"
  Demux/3 -> BusCreator/3  "PTC_Cfg nMotor"
  Demux/4 -> BusCreator/4  "PTC_Cfg nGearBoxM"
  Demux/5 -> BusCreator/5  "PTC_Cfg nPlanetGear"
  Demux/6 -> BusCreator/6  "PTC_Cfg Vehicle_nWheels"
  Demux/7 -> BusCreator/7  "PTC_Cfg WheelRadius"
  Demux/8 -> BusCreator/8  "PTC_Cfg Aero_Frcx"
  Demux/9 -> BusCreator/9  "PTC_Cfg DL_iDiff_mean"
  Demux/10 -> BusCreator/10  "PTC_Cfg DriveSourcePos0"
  Demux/11 -> BusCreator/11  "PTC_Cfg DriveSourcePos1"
  Demux/12 -> BusCreator/12  "PTC_Cfg DriveSourcePos2"
  Demux/13 -> BusCreator/13  "PTC_Cfg DriveSourcePos3"

== system TorqueVect/CarMaker/IPG Vehicle/PowerTrain/PTControl Example/PTControl_In/CreateBus PTC_Cfg Motor ==
  In : Inport
  BusCreator : BusCreator  Inputs=16
  Demux : Demux  Outputs=16
      settings: DisplayOption=none
  Out : Outport  VectorParamsAs1DForOutWhenUnconnected=off
  wires:
  In/1 -> Demux/1
  BusCreator/1 -> Out/1
  Demux/1 -> BusCreator/1  "PTC_Cfg Motor0 Level"
  Demux/2 -> BusCreator/2  "PTC_Cfg Motor0 Ratio"
  Demux/3 -> BusCreator/3  "PTC_Cfg Motor0 rotv_Mot_max"
  Demux/4 -> BusCreator/4  "PTC_Cfg Motor0 rotv_Gen_max"
  Demux/5 -> BusCreator/5  "PTC_Cfg Motor1 Level"
  Demux/6 -> BusCreator/6  "PTC_Cfg Motor1 Ratio"
  Demux/7 -> BusCreator/7  "PTC_Cfg Motor1 rotv_Mot_max"
  Demux/8 -> BusCreator/8  "PTC_Cfg Motor1 rotv_Gen_max"
  Demux/9 -> BusCreator/9  "PTC_Cfg Motor2 Level"
  Demux/10 -> BusCreator/10  "PTC_Cfg Motor2 Ratio"
  Demux/11 -> BusCreator/11  "PTC_Cfg Motor2 rotv_Mot_max"
  Demux/12 -> BusCreator/12  "PTC_Cfg Motor2 rotv_Gen_max"
  Demux/13 -> BusCreator/13  "PTC_Cfg Motor3 Level"
  Demux/14 -> BusCreator/14  "PTC_Cfg Motor3 Ratio"
  Demux/15 -> BusCreator/15  "PTC_Cfg Motor3 rotv_Mot_max"
  Demux/16 -> BusCreator/16  "PTC_Cfg Motor3 rotv_Gen_max"

== system TorqueVect/CarMaker/IPG Vehicle/PowerTrain/PTControl Example/PTControl_In/CreateBus PTC_Cfg PlanetGear ==
  In : Inport
  BusCreator : BusCreator  Inputs=1
  Demux : Demux  Outputs=1
      settings: DisplayOption=none
  Out : Outport  VectorParamsAs1DForOutWhenUnconnected=off
  wires:
  In/1 -> Demux/1
  BusCreator/1 -> Out/1
  Demux/1 -> BusCreator/1  "PTC_Cfg PlanetGear0 Ratio"

== system TorqueVect/CarMaker/IPG Vehicle/PowerTrain/PTControl Example/PTControl/Torque Control 0/Electronic Gas Pedal FL ==
  TV_On : Inport
  VC.Gas : Inport  Port=2
  Define CM Dict : CarMaker4SL/Define CM Dict  xname=E_Gas_FL  xmono=off  xtype=Double4  xdvaplace=None  xnstates=0  xfirststate=0  xinitial=0
  Read CM Dict : CarMaker4SL/Read CM Dict  xname=E_Gas_FL  xsync=off  xstime=Continuous
  Read CM Dict1 : CarMaker4SL/Read CM Dict  xname=Car.LongSlipFL  xsync=off  xstime=Continuous
  Switch : Switch  Criteria=u2 > Threshold
  Traction Control FL : Subsystem
  Write CM Dict : CarMaker4SL/Write CM Dict  xname=E_Gas_FL  xsync=off
  Motor_Gas_FL : Outport  VectorParamsAs1DForOutWhenUnconnected=off
  wires:
  Read CM Dict/1 -> Traction Control FL/2(E_Gas.)
  Read CM Dict1/1 -> Traction Control FL/3(Car.LongSlip)
  VC.Gas/1 -> Switch/3, Traction Control FL/1(VC.Gas)
  Switch/1 -> Motor_Gas_FL/1
  TV_On/1 -> Switch/2
  Traction Control FL/1(E_Gas) -> Switch/1, Write CM Dict/1

== system TorqueVect/CarMaker/IPG Vehicle/PowerTrain/PTControl Example/PTControl/Torque Control 0/Torque Vectoring FL ==
  Abs : Abs
  Abs2 : Abs
  Constant : Constant
  Divide : Product  Inputs=*/
  Gain : Gain  Gain=-1
  Gravity : Gain  Gain=9.81
  Lookup Table : Lookup  InputValues=[0,0.1,0.2,0.3,0.4,0.5,0.6,0.7,0.8,1,2,3,4]  Table=[0,0,0.05,0.1,0.2,0.3,0.4,0.5,0.6,0.7,1,1,1]
  Override : Gain  Gain=TV_Override
  Product : Product  RndMeth=Zero
  Read CM Dict : CarMaker4SL/Read CM Dict  xname=Car.muRoadFL  xsync=off  xstime=Continuous
  Read CM Dict1 : CarMaker4SL/Read CM Dict  xname=Car.v  xsync=off  xstime=Continuous
  Read CM Dict2 : CarMaker4SL/Read CM Dict  xname=Car.YawRate  xsync=off  xstime=Continuous
  Read CM Dict3 : CarMaker4SL/Read CM Dict  xname=VC.Steer.Ang  xsync=off  xstime=Continuous
  Subtract : Sum  Inputs=+-
  Switch : Switch  Criteria=u2 > Threshold
  TV FL : Outport  VectorParamsAs1DForOutWhenUnconnected=off
  wires:
  Gain/1 -> Lookup Table/1
  Abs2/1 -> Subtract/2
  Lookup Table/1 -> Product/2
  Read CM Dict3/1 -> Gain/1
  Product/1 -> TV FL/1
  Subtract/1 -> Product/1
  Read CM Dict2/1 -> Abs2/1
  Divide/1 -> Subtract/1
  Abs/1 -> Divide/2
  Switch/1 -> Abs/1
  Constant/1 -> Switch/3
  Read CM Dict1/1 -> Switch/2, Switch/1
  Override/1 -> Divide/1
  Gravity/1 -> Override/1
  Read CM Dict/1 -> Gravity/1

== system TorqueVect/CarMaker/IPG Vehicle/PowerTrain/PTControl Example/PTControl/Torque Control 1/Electronic Gas Pedal FR ==
  TV_On : Inport
  VC.Gas : Inport  Port=2
  Define CM Dict : CarMaker4SL/Define CM Dict  xname=E_Gas_FR  xmono=off  xtype=Double4  xdvaplace=None  xnstates=0  xfirststate=0  xinitial=0
  Read CM Dict : CarMaker4SL/Read CM Dict  xname=E_Gas_FR  xsync=off  xstime=Continuous
  Read CM Dict1 : CarMaker4SL/Read CM Dict  xname=Car.LongSlipFR  xsync=off  xstime=Continuous
  Switch : Switch  Criteria=u2 > Threshold
  Traction Control FR : Subsystem
  Write CM Dict : CarMaker4SL/Write CM Dict  xname=E_Gas_FR  xsync=off
  Motor_Gas_FR : Outport  VectorParamsAs1DForOutWhenUnconnected=off
  wires:
  Traction Control FR/1(E_Gas) -> Write CM Dict/1, Switch/1
  TV_On/1 -> Switch/2
  Switch/1 -> Motor_Gas_FR/1
  VC.Gas/1 -> Traction Control FR/1(VC.Gas), Switch/3
  Read CM Dict1/1 -> Traction Control FR/3(Car.LongSlip)
  Read CM Dict/1 -> Traction Control FR/2(E_Gas.)

== system TorqueVect/CarMaker/IPG Vehicle/PowerTrain/PTControl Example/PTControl/Torque Control 1/Torque Vectoring FR ==
  Abs : Abs
  Abs2 : Abs
  Constant : Constant
  Divide : Product  Inputs=*/
  Gain : Gain  Gain=-1
  Gravity : Gain  Gain=9.81
  Lookup Table : Lookup  InputValues=[0,0.1,0.2,0.3,0.4,0.5,0.6,0.7,0.8,1,2,3,4]  Table=[0,0,0.05,0.1,0.2,0.3,0.4,0.5,0.6,0.7,1,1,1]
  Override : Gain  Gain=TV_Override
  Product : Product  RndMeth=Zero
  Read CM Dict : CarMaker4SL/Read CM Dict  xname=Car.muRoadFR  xsync=off  xstime=Continuous
  Read CM Dict1 : CarMaker4SL/Read CM Dict  xname=Car.v  xsync=off  xstime=Continuous
  Read CM Dict2 : CarMaker4SL/Read CM Dict  xname=Car.YawRate  xsync=off  xstime=Continuous
  Read CM Dict3 : CarMaker4SL/Read CM Dict  xname=VC.Steer.Ang  xsync=off  xstime=Continuous
  Subtract : Sum  Inputs=+-
  Switch : Switch  Criteria=u2 > Threshold
  TV FR : Outport  VectorParamsAs1DForOutWhenUnconnected=off
  wires:
  Read CM Dict/1 -> Gravity/1
  Gravity/1 -> Override/1
  Override/1 -> Divide/1
  Read CM Dict1/1 -> Switch/1, Switch/2
  Constant/1 -> Switch/3
  Switch/1 -> Abs/1
  Abs/1 -> Divide/2
  Divide/1 -> Subtract/1
  Read CM Dict2/1 -> Abs2/1
  Subtract/1 -> Product/1
  Product/1 -> TV FR/1
  Read CM Dict3/1 -> Gain/1
  Lookup Table/1 -> Product/2
  Abs2/1 -> Subtract/2
  Gain/1 -> Lookup Table/1

== system TorqueVect/CarMaker/IPG Vehicle/PowerTrain/PTControl Example/PTControl/Torque Control 2/Electronic Gas Pedal RL ==
  TV_On : Inport
  VC.Gas : Inport  Port=2
  Define CM Dict : CarMaker4SL/Define CM Dict  xname=E_Gas_RL  xmono=off  xtype=Double4  xdvaplace=None  xnstates=0  xfirststate=0  xinitial=0
  Read CM Dict : CarMaker4SL/Read CM Dict  xname=E_Gas_RL  xsync=off  xstime=Continuous
  Read CM Dict1 : CarMaker4SL/Read CM Dict  xname=Car.LongSlipRL  xsync=off  xstime=Continuous
  Switch : Switch  Criteria=u2 > Threshold
  Traction Control RL : Subsystem
  Write CM Dict : CarMaker4SL/Write CM Dict  xname=E_Gas_RL  xsync=off
  Motor_Gas_RL : Outport  VectorParamsAs1DForOutWhenUnconnected=off
  wires:
  Traction Control RL/1(E_Gas) -> Write CM Dict/1, Switch/1
  TV_On/1 -> Switch/2
  Switch/1 -> Motor_Gas_RL/1
  VC.Gas/1 -> Traction Control RL/1(VC.Gas), Switch/3
  Read CM Dict1/1 -> Traction Control RL/3(Car.LongSlip)
  Read CM Dict/1 -> Traction Control RL/2(E_Gas.)

== system TorqueVect/CarMaker/IPG Vehicle/PowerTrain/PTControl Example/PTControl/Torque Control 2/Torque Vectoring RL ==
  Abs : Abs
  Abs2 : Abs
  Constant : Constant
  Divide : Product  Inputs=*/
  Gain : Gain  Gain=-1
  Gravity : Gain  Gain=9.81
  Lookup Table : Lookup  InputValues=[0,0.1,0.2,0.3,0.4,0.5,0.6,0.7,0.8,1,2,3,4]  Table=[0,0,0.05,0.1,0.2,0.3,0.4,0.5,0.6,0.7,1,1,1]
  Override : Gain  Gain=TV_Override
  Product : Product  RndMeth=Zero
  Read CM Dict : CarMaker4SL/Read CM Dict  xname=Car.muRoadRL  xsync=off  xstime=Continuous
  Read CM Dict1 : CarMaker4SL/Read CM Dict  xname=Car.v  xsync=off  xstime=Continuous
  Read CM Dict2 : CarMaker4SL/Read CM Dict  xname=Car.YawRate  xsync=off  xstime=Continuous
  Read CM Dict3 : CarMaker4SL/Read CM Dict  xname=VC.Steer.Ang  xsync=off  xstime=Continuous
  Subtract : Sum  Inputs=+-
  Switch : Switch  Criteria=u2 > Threshold
  TV RL : Outport  VectorParamsAs1DForOutWhenUnconnected=off
  wires:
  Read CM Dict/1 -> Gravity/1
  Gravity/1 -> Override/1
  Override/1 -> Divide/1
  Read CM Dict1/1 -> Switch/1, Switch/2
  Constant/1 -> Switch/3
  Switch/1 -> Abs/1
  Abs/1 -> Divide/2
  Divide/1 -> Subtract/1
  Read CM Dict2/1 -> Abs2/1
  Subtract/1 -> Product/1
  Product/1 -> TV RL/1
  Read CM Dict3/1 -> Gain/1
  Lookup Table/1 -> Product/2
  Abs2/1 -> Subtract/2
  Gain/1 -> Lookup Table/1

== system TorqueVect/CarMaker/IPG Vehicle/PowerTrain/PTControl Example/PTControl/Torque Control 3/Electronic Gas Pedal RR ==
  TV_On : Inport
  VC.Gas : Inport  Port=2
  Define CM Dict : CarMaker4SL/Define CM Dict  xname=E_Gas_RR  xmono=off  xtype=Double4  xdvaplace=None  xnstates=0  xfirststate=0  xinitial=0
  Read CM Dict : CarMaker4SL/Read CM Dict  xname=E_Gas_RR  xsync=off  xstime=Continuous
  Read CM Dict1 : CarMaker4SL/Read CM Dict  xname=Car.LongSlipRR  xsync=off  xstime=Continuous
  Switch : Switch  Criteria=u2 > Threshold
  Traction Control RR : Subsystem
  Write CM Dict : CarMaker4SL/Write CM Dict  xname=E_Gas_RR  xsync=off
  Motor_Gas_RR : Outport  VectorParamsAs1DForOutWhenUnconnected=off
  wires:
  Read CM Dict/1 -> Traction Control RR/2(E_Gas.)
  Read CM Dict1/1 -> Traction Control RR/3(Car.LongSlip)
  VC.Gas/1 -> Switch/3, Traction Control RR/1(VC.Gas)
  Switch/1 -> Motor_Gas_RR/1
  TV_On/1 -> Switch/2
  Traction Control RR/1(E_Gas) -> Switch/1, Write CM Dict/1

== system TorqueVect/CarMaker/IPG Vehicle/PowerTrain/PTControl Example/PTControl/Torque Control 3/Torque Vectoring RR ==
  Abs : Abs
  Abs2 : Abs
  Constant : Constant
  Divide : Product  Inputs=*/
  Gain : Gain  Gain=-1
  Gravity : Gain  Gain=9.81
  Lookup Table : Lookup  InputValues=[0,0.1,0.2,0.3,0.4,0.5,0.6,0.7,0.8,1,2,3,4]  Table=[0,0,0.05,0.1,0.2,0.3,0.4,0.5,0.6,0.7,1,1,1]
  Override : Gain  Gain=TV_Override
  Product : Product  RndMeth=Zero
  Read CM Dict : CarMaker4SL/Read CM Dict  xname=Car.muRoadRR  xsync=off  xstime=Continuous
  Read CM Dict1 : CarMaker4SL/Read CM Dict  xname=Car.v  xsync=off  xstime=Continuous
  Read CM Dict2 : CarMaker4SL/Read CM Dict  xname=Car.YawRate  xsync=off  xstime=Continuous
  Read CM Dict3 : CarMaker4SL/Read CM Dict  xname=VC.Steer.Ang  xsync=off  xstime=Continuous
  Subtract : Sum  Inputs=+-
  Switch : Switch  Criteria=u2 > Threshold
  TV RR : Outport  VectorParamsAs1DForOutWhenUnconnected=off
  wires:
  Gain/1 -> Lookup Table/1
  Abs2/1 -> Subtract/2
  Lookup Table/1 -> Product/2
  Read CM Dict3/1 -> Gain/1
  Product/1 -> TV RR/1
  Subtract/1 -> Product/1
  Read CM Dict2/1 -> Abs2/1
  Divide/1 -> Subtract/1
  Abs/1 -> Divide/2
  Switch/1 -> Abs/1
  Constant/1 -> Switch/3
  Read CM Dict1/1 -> Switch/2, Switch/1
  Override/1 -> Divide/1
  Gravity/1 -> Override/1
  Read CM Dict/1 -> Gravity/1

== system TorqueVect/CarMaker/IPG Vehicle/PowerTrain/PTControl Example/PTControl/Torque Control 0/Electronic Gas Pedal FL/Traction Control FL ==
  VC.Gas : Inport
  E_Gas. : Inport  Port=2
  Car.LongSlip : Inport  Port=3
  Add : Sum
  Compare To Constant : simulink/Logic and Bit Operations/Compare To Constant  relop=>  const=TC_Derivative  OutDataTypeStr=uint8  ZeroCross=off
  Derivative : Derivative
  Fcn : Fcn  Expr=u >0.05
  Fcn1 : Fcn  Expr=u+TC_Incr_Gas
  Fcn2 : Fcn  Expr=u-TC_Decr_Gas
  Multiport Switch : MultiPortSwitch  DataPortOrder=Zero-based contiguous  zeroidx=on
  Relational Operator : RelationalOperator  Operator=<=  RndMeth=Nearest
  Relay : Relay  OnSwitchValue=TC_Relay_On  OffSwitchValue=TC_Relay_Off
  S-R Flip-Flop : simulink_extras/Flip Flops/S-R Flip-Flop  initial_condition=0
  Saturation : Saturate  UpperLimit=1  LowerLimit=0
  Saturation1 : Saturate  UpperLimit=1  LowerLimit=0
  Switch : Switch  Criteria=u2 > Threshold
  Terminator : Terminator
  E_Gas : Outport  VectorParamsAs1DForOutWhenUnconnected=off
  wires:
  [A] -> Switch/3
  Saturation/1 -> Multiport Switch/4
  Fcn2/1 -> Saturation/1
  Saturation1/1 -> Switch/1
  Fcn1/1 -> Saturation1/1
  Relational Operator/1 -> S-R Flip-Flop/2
  Fcn/1 -> S-R Flip-Flop/1
  Switch/1 -> Multiport Switch/2
  S-R Flip-Flop/1 -> Switch/2
  S-R Flip-Flop/2 -> Terminator/1
  E_Gas./1 -> Multiport Switch/3, Fcn2/1, Fcn1/1, Relational Operator/2
  VC.Gas/1 -> [A], Relational Operator/1
  Multiport Switch/1 -> E_Gas/1
  Add/1 -> Multiport Switch/1
  Compare To Constant/1 -> Add/2
  Derivative/1 -> Compare To Constant/1
  Relay/1 -> Add/1
  Car.LongSlip/1 -> Fcn/1, Derivative/1, Relay/1

== system TorqueVect/CarMaker/IPG Vehicle/PowerTrain/PTControl Example/PTControl/Torque Control 1/Electronic Gas Pedal FR/Traction Control FR ==
  VC.Gas : Inport
  E_Gas. : Inport  Port=2
  Car.LongSlip : Inport  Port=3
  Add : Sum
  Compare To Constant : simulink/Logic and Bit Operations/Compare To Constant  relop=>  const=TC_Derivative  OutDataTypeStr=uint8  ZeroCross=off
  Derivative : Derivative
  Fcn : Fcn  Expr=u >0.05
  Fcn1 : Fcn  Expr=u+TC_Incr_Gas
  Fcn2 : Fcn  Expr=u-TC_Decr_Gas
  Multiport Switch : MultiPortSwitch  DataPortOrder=Zero-based contiguous  zeroidx=on
  Relational Operator : RelationalOperator  Operator=<=  RndMeth=Nearest
  Relay : Relay  OnSwitchValue=TC_Relay_On  OffSwitchValue=TC_Relay_Off
  S-R Flip-Flop : simulink_extras/Flip Flops/S-R Flip-Flop  initial_condition=0
  Saturation : Saturate  UpperLimit=1  LowerLimit=0
  Saturation1 : Saturate  UpperLimit=1  LowerLimit=0
  Switch : Switch  Criteria=u2 > Threshold
  Terminator : Terminator
  E_Gas : Outport  VectorParamsAs1DForOutWhenUnconnected=off
  wires:
  Car.LongSlip/1 -> Relay/1, Derivative/1, Fcn/1
  Relay/1 -> Add/1
  Derivative/1 -> Compare To Constant/1
  Compare To Constant/1 -> Add/2
  Add/1 -> Multiport Switch/1
  Multiport Switch/1 -> E_Gas/1
  VC.Gas/1 -> Relational Operator/1, [A]
  E_Gas./1 -> Relational Operator/2, Fcn1/1, Fcn2/1, Multiport Switch/3
  S-R Flip-Flop/2 -> Terminator/1
  S-R Flip-Flop/1 -> Switch/2
  Switch/1 -> Multiport Switch/2
  Fcn/1 -> S-R Flip-Flop/1
  Relational Operator/1 -> S-R Flip-Flop/2
  Fcn1/1 -> Saturation1/1
  Saturation1/1 -> Switch/1
  Fcn2/1 -> Saturation/1
  Saturation/1 -> Multiport Switch/4
  [A] -> Switch/3

== system TorqueVect/CarMaker/IPG Vehicle/PowerTrain/PTControl Example/PTControl/Torque Control 2/Electronic Gas Pedal RL/Traction Control RL ==
  VC.Gas : Inport
  E_Gas. : Inport  Port=2
  Car.LongSlip : Inport  Port=3
  Add : Sum
  Compare To Constant : simulink/Logic and Bit Operations/Compare To Constant  relop=>  const=TC_Derivative  OutDataTypeStr=uint8  ZeroCross=off
  Derivative : Derivative
  Fcn : Fcn  Expr=u >0.05
  Fcn1 : Fcn  Expr=u+TC_Incr_Gas
  Fcn2 : Fcn  Expr=u-TC_Decr_Gas
  Multiport Switch : MultiPortSwitch  DataPortOrder=Zero-based contiguous  zeroidx=on
  Relational Operator : RelationalOperator  Operator=<=  RndMeth=Nearest
  Relay : Relay  OnSwitchValue=TC_Relay_On  OffSwitchValue=TC_Relay_Off
  S-R Flip-Flop : simulink_extras/Flip Flops/S-R Flip-Flop  initial_condition=0
  Saturation : Saturate  UpperLimit=1  LowerLimit=0
  Saturation1 : Saturate  UpperLimit=1  LowerLimit=0
  Switch : Switch  Criteria=u2 > Threshold
  Terminator : Terminator
  E_Gas : Outport  VectorParamsAs1DForOutWhenUnconnected=off
  wires:
  Car.LongSlip/1 -> Relay/1, Derivative/1, Fcn/1
  Relay/1 -> Add/1
  Derivative/1 -> Compare To Constant/1
  Compare To Constant/1 -> Add/2
  Add/1 -> Multiport Switch/1
  Multiport Switch/1 -> E_Gas/1
  VC.Gas/1 -> Relational Operator/1, [A]
  E_Gas./1 -> Relational Operator/2, Fcn1/1, Fcn2/1, Multiport Switch/3
  S-R Flip-Flop/2 -> Terminator/1
  S-R Flip-Flop/1 -> Switch/2
  Switch/1 -> Multiport Switch/2
  Fcn/1 -> S-R Flip-Flop/1
  Relational Operator/1 -> S-R Flip-Flop/2
  Fcn1/1 -> Saturation1/1
  Saturation1/1 -> Switch/1
  Fcn2/1 -> Saturation/1
  Saturation/1 -> Multiport Switch/4
  [A] -> Switch/3

== system TorqueVect/CarMaker/IPG Vehicle/PowerTrain/PTControl Example/PTControl/Torque Control 3/Electronic Gas Pedal RR/Traction Control RR ==
  VC.Gas : Inport
  E_Gas. : Inport  Port=2
  Car.LongSlip : Inport  Port=3
  Add : Sum
  Compare To Constant : simulink/Logic and Bit Operations/Compare To Constant  relop=>  const=TC_Derivative  OutDataTypeStr=uint8  ZeroCross=off
  Derivative : Derivative
  Fcn : Fcn  Expr=u >0.05
  Fcn1 : Fcn  Expr=u+TC_Incr_Gas
  Fcn2 : Fcn  Expr=u-TC_Decr_Gas
  Multiport Switch : MultiPortSwitch  DataPortOrder=Zero-based contiguous  zeroidx=on
  Relational Operator : RelationalOperator  Operator=<=  RndMeth=Nearest
  Relay : Relay  OnSwitchValue=TC_Relay_On  OffSwitchValue=TC_Relay_Off
  S-R Flip-Flop : simulink_extras/Flip Flops/S-R Flip-Flop  initial_condition=0
  Saturation : Saturate  UpperLimit=1  LowerLimit=0
  Saturation1 : Saturate  UpperLimit=1  LowerLimit=0
  Switch : Switch  Criteria=u2 > Threshold
  Terminator : Terminator
  E_Gas : Outport  VectorParamsAs1DForOutWhenUnconnected=off
  wires:
  [A] -> Switch/3
  Saturation/1 -> Multiport Switch/4
  Fcn2/1 -> Saturation/1
  Saturation1/1 -> Switch/1
  Fcn1/1 -> Saturation1/1
  Relational Operator/1 -> S-R Flip-Flop/2
  Fcn/1 -> S-R Flip-Flop/1
  Switch/1 -> Multiport Switch/2
  S-R Flip-Flop/1 -> Switch/2
  S-R Flip-Flop/2 -> Terminator/1
  E_Gas./1 -> Multiport Switch/3, Fcn2/1, Fcn1/1, Relational Operator/2
  VC.Gas/1 -> [A], Relational Operator/1
  Multiport Switch/1 -> E_Gas/1
  Add/1 -> Multiport Switch/1
  Compare To Constant/1 -> Add/2
  Derivative/1 -> Compare To Constant/1
  Relay/1 -> Add/1
  Car.LongSlip/1 -> Fcn/1, Derivative/1, Relay/1
